simulink model "openloop501_sim"  (R2022a)
settings: Solver=ode23s  StartTime=0.0  StopTime=2000  RelTol=1e-3
settings Model: Creator=danie  LastModifiedBy=danie

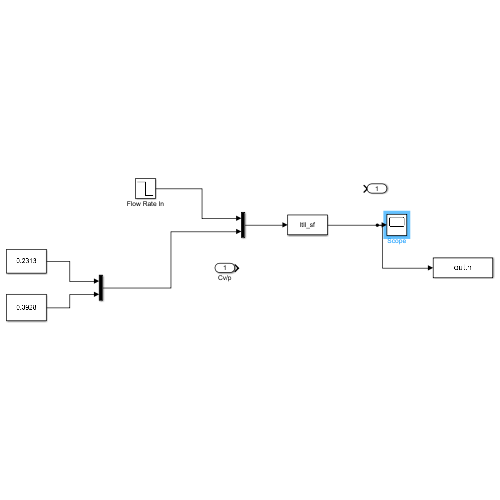
[thumbnail: Simulink's stored preview of the top-level diagram]
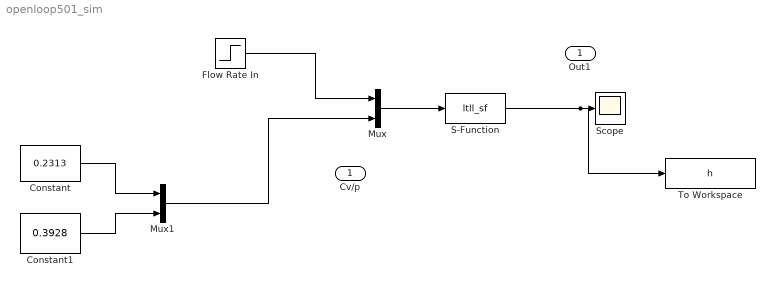
== system openloop501_sim ==
  Cv/p : Inport
  Constant : Constant  Value=0.2313
  Constant1 : Constant  Value=0.3928
  Flow Rate In : Step  Time=0  Before=2.65  After=1.6  SampleTime=0
  Mux : Mux  Inputs=2
  Mux1 : Mux  Inputs=2
  S-Function : S-Function  FunctionName=ltll_sf  SFunctionDeploymentMode=off  EnableBusSupport=off
  Scope : Scope
  To Workspace : ToWorkspace  VariableName=h  SampleTime=-1
  Out1 : Outport
  wires:
  S-Function/1 -> To Workspace/1, Scope/1
  Flow Rate In/1 -> Mux/1
  Mux/1 -> S-Function/1
  Constant/1 -> Mux1/1
  Constant1/1 -> Mux1/2
  Mux1/1 -> Mux/2
